simulink library "calc_B_FandMaero"  (R2020a)
settings: Solver=VariableStepAuto  StartTime=0.0  StopTime=10.0  RelTol=1e-3
undefined symbols (not defined in the file): AoA_vals, CD_vals, CL_vals, rho, Sref
libraries: vrlib x6, calcCLandCD x1, calcDynamicPressure x1
settings Model: Creator=Ayaz  LastModifiedBy=Ayaz

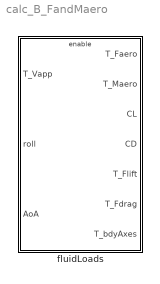
== system calc_B_FandMaero ==
  fluidLoads : Subsystem  mask{refArea=Sref, aeroCent=[-1;0;0], flowDensity=rho, AoA_vals=AoA_vals, CL_vals=CL_vals, CD_vals=CD_vals}
      mask prompts: refArea "Reference area [m^2]"; aeroCent "Aerodynamic center [m]"; flowDensity "Flow density [kg/m^3]"; AoA_vals "Angle of attack values [deg]"; CL_vals "Lift coeffcient values [-]"; CD_vals "Drag coefficient values [-]"
      mask TypeOptions flowDensity: dynamicPressure/flowDensity
      mask TypeOptions AoA_vals: CLandCD/AoA_vals
      mask TypeOptions CL_vals: CLandCD/CL_vals
      mask TypeOptions CD_vals: CLandCD/CD_vals

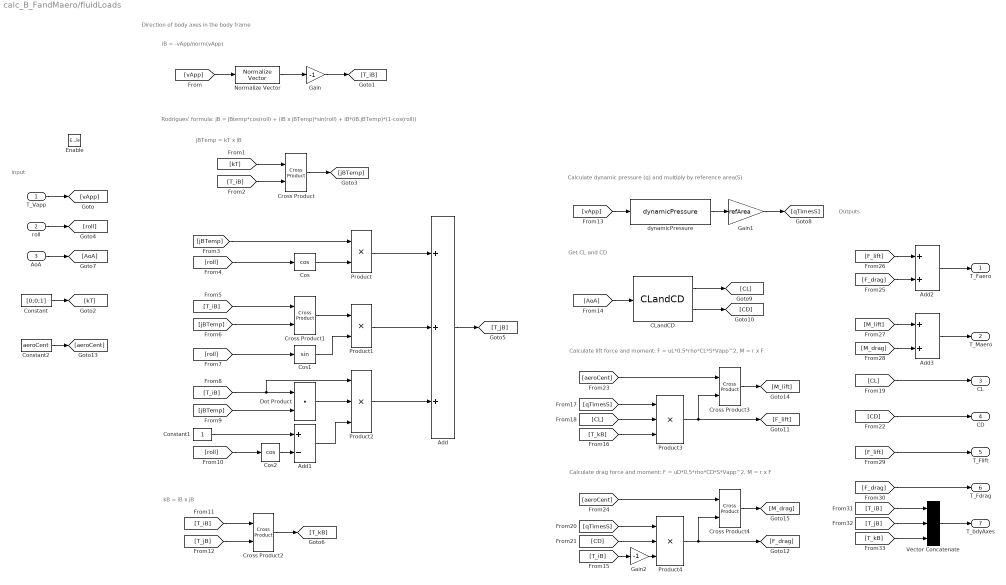
== system calc_B_FandMaero/fluidLoads ==
  note: Outputs
  note: Get CL and CD
  note: Calculate dynamic pressure (q) and multiply by reference area(S)
  note: Direction of body axes in the body frame
  note: jBTemp = kT x iB
  note: Rodrigues' formula: jB = jBtemp*cos(roll) + (iB x jBTemp)*sin(roll) + iB*(iB.jBTemp)*(1-cos(roll))
  note: iB = -vApp/norm(vApp)
  note: input
  note: kB = iB x jB
  note: Calculate lift force and moment: F = uL*0.5*rho*CL*S*Vapp^2, M = r x F
  note: Calculate drag force and moment: F = uD*0.5*rho*CD*S*Vapp^2, M = r x F
  T_Vapp : Inport
  roll : Inport  Port=2
  AoA : Inport  Port=3
  Enable : EnablePort
  Add : Sum  Inputs=+++
  Add1 : Sum  Inputs=+-
  Add2 : Sum
  Add3 : Sum
  CLandCD : calcCLandCD/CLandCD  AoA_vals=AoA_vals  CL_vals=CL_vals  CD_vals=CD_vals
  Constant : Constant  Value=[0;0;1]  VectorParams1D=off
  Constant1 : Constant
  Constant2 : Constant  Value=aeroCent  VectorParams1D=off
  Cos : Trigonometry  Operator=cos
  Cos1 : Trigonometry
  Cos2 : Trigonometry  Operator=cos
  Cross Product{,1..4} (5 alike) : vrlib/Utilities/Cross Product
  Dot Product : DotProduct  InputSameDT=on  OutDataTypeStr=Inherit: Inherit via internal rule
  Gain : Gain  Gain=-1
  Gain1 : Gain  Gain=refArea
  Gain2 : Gain  Gain=-1
  Normalize Vector : vrlib/Utilities/Normalize Vector  maxzero=0
  Product : Product
  Product1 : Product
  Product2 : Product  Inputs=3
  Product3 : Product  Inputs=3
  Product4 : Product  Inputs=3
  Vector Concatenate : Concatenate  NumInputs=3  Mode=Multidimensional array  ConcatenateDimension=2
  dynamicPressure : calcDynamicPressure/dynamicPressure  flowDensity=flowDensity
  T_Faero : Outport
  T_Maero : Outport  Port=2
  CL : Outport  Port=3
  CD : Outport  Port=4
  T_Flift : Outport  Port=5
  T_Fdrag : Outport  Port=6
  T_bdyAxes : Outport  Port=7
  wires:
  Gain2/1 -> Product4/3
  [T_iB] -> Gain2/1
  T_Vapp/1 -> [vApp]
  [vApp] -> Normalize Vector/1
  Normalize Vector/1 -> Gain/1
  Gain/1 -> [T_iB]
  Constant/1 -> [kT]
  [kT] -> Cross Product/1
  [T_iB] -> Cross Product/2
  Cross Product/1 -> [jBTemp]
  roll/1 -> [roll]
  [jBTemp] -> Product/1
  [roll] -> Cos/1
  Cos/1 -> Product/2
  Product/1 -> Add/1
  [T_iB] -> Cross Product1/1
  [jBTemp] -> Cross Product1/2
  Cross Product1/1 -> Product1/1
  Cos1/1 -> Product1/2
  [roll] -> Cos1/1
  Product1/1 -> Add/2
  [T_iB] -> Product2/1, Dot Product/1
  [jBTemp] -> Dot Product/2
  Dot Product/1 -> Product2/2
  [roll] -> Cos2/1
  Cos2/1 -> Add1/2
  Constant1/1 -> Add1/1
  Add1/1 -> Product2/3
  Product2/1 -> Add/3
  Add/1 -> [T_jB]
  Cross Product2/1 -> [T_kB]
  [T_jB] -> Cross Product2/2
  [T_iB] -> Cross Product2/1
  AoA/1 -> [AoA]
  [vApp] -> dynamicPressure/1
  [AoA] -> CLandCD/1
  dynamicPressure/1 -> Gain1/1
  Gain1/1 -> [qTimesS]
  CLandCD/2 -> [CD]
  CLandCD/1 -> [CL]
  [qTimesS] -> Product3/1
  [CL] -> Product3/2
  [T_kB] -> Product3/3
  [CD] -> Product4/2
  [CL] -> CL/1
  [CD] -> CD/1
  Product3/1 -> Cross Product3/2, [F_lift]
  Constant2/1 -> [aeroCent]
  [aeroCent] -> Cross Product3/1
  Cross Product3/1 -> [M_lift]
  Cross Product4/1 -> [M_drag]
  [aeroCent] -> Cross Product4/1
  Product4/1 -> [F_drag], Cross Product4/2
  [qTimesS] -> Product4/1
  [F_drag] -> Add2/2
  [F_lift] -> Add2/1
  Add2/1 -> T_Faero/1
  Add3/1 -> T_Maero/1
  [M_lift] -> Add3/1
  [M_drag] -> Add3/2
  [F_lift] -> T_Flift/1
  [F_drag] -> T_Fdrag/1
  [T_iB] -> Vector Concatenate/1
  [T_jB] -> Vector Concatenate/2
  [T_kB] -> Vector Concatenate/3
  Vector Concatenate/1 -> T_bdyAxes/1
